simulink model "untitled"  (R2021a)
settings: Solver=VariableStepAuto  StartTime=0.0  StopTime=5  RelTol=1e-3
settings Model: Creator=Administrator  LastModifiedBy=Administrator

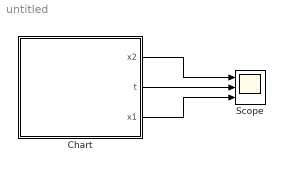
== system untitled ==
  Chart : Stateflow chart  TreatAsAtomicUnit=on
  Scope : Scope  NumInputPorts=3
  wires:
  Chart/3(x1) -> Scope/3
  Chart/1(x2) -> Scope/1
  Chart/2(t) -> Scope/2

== stateflow chart untitled/Chart ==
  state q1
    entry:
    t=0;
    v1=1/2;
    v2=-1/2;
    during:
    t=t+0.01;
    x1=x1_0+v1*t;
    x2=x2_0+v2*t;
    exit:
    x1_0=x1;
    x2_0=x2;
    t=0;
  state q2
    entry:
    t=0;
    v1=-1/2;
    v2=1/2;
    during:
    t=t+0.01;
    x1=x1_0+v1*t;
    x2=x2_0+v2*t;
    exit:
    x1_0=x1;
    x2_0=x2;
    t=0;
  (default) -> q1 : {x1=1;
      | x2=1;
      | x1_0=0;
      | x2_0=1;}
  q2 -> q1 : [x1<=0]
  q1 -> q2 : [x2<=0]
  data: x2 output; t output; x1 output; v1 local; v2 local; x1_0 local; x2_0 local
